simulink model "learned_HA0"  (R2022b)
settings: Solver=FixedStepAuto  StartTime=0.0  StopTime=timeFinal  FixedStep=timeStepMax  RelTol=1e-3
undefined symbols (not defined in the file): a1, a2
settings Model: Creator=jun  LastModifiedBy=jun

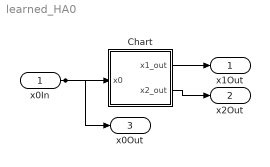
== system learned_HA0 ==
  x0In : Inport
  Chart : Stateflow chart  TreatAsAtomicUnit=on
  x1Out : Outport  SignalName=x1Out
  x2Out : Outport  Port=2  SignalName=x2Out
  x0Out : Outport  Port=3  SignalName=x0Out
  wires:
  Chart/2(x2_out) -> x2Out/1
  Chart/1(x1_out) -> x1Out/1
  x0In/1 -> x0Out/1, Chart/1(x0)

== stateflow chart learned_HA0/Chart ==
  settings: updateMethod=CONTINUOUS  executeAtInitialization=1
  state loc1
    du:
    x1_dot = x0 * 2.1894941703248746e-09 + x1 * 3.311445284648329e-10 + x2 * 0.9999999993832541 + 2.205176730107894e-08;
    x2_dot = x0 * 1.0000002537439894 + x1 * 1.3012050788811615e-08 + x2 * -6.066488462071542e-08 + 2.742040890983218e-06;
    exit:
    x1_out = x1;
    x2_out = x2;
  (junction 2) -> loc1 : [x0 * -0.000614101399950075 + x1 * 7.1072164927641275 + x2 * 0.002028184397089736 + -0.6595328211966963 <= 0]{x1 = x0 * 0.0 + x1 * 0.0 + x2 * 0.0 + 0.0; x2 = x0 * -2.1616467629052686e-14 + x1 * -3.7625458304546555e-13 + x2 * -0.7999999999999966 + -1.9451107391432743e-13; }
  (default) -> loc1 : { x1 = a1; x2 = a2; }
  loc1 -> (junction 5) [order 2]
  (junction 5) -> loc1 : { x1 = x1; x2 = x2; }
  loc1 -> (junction 2) [order 1]
  data: x0 input; x1_out output; x2_out output; x1 local double; x2 local double; a1 parameter; a2 parameter
  data x1 settings: updateMethod=SF_CONTINUOUS_TIME_DATA
  data x2 settings: updateMethod=SF_CONTINUOUS_TIME_DATA
